simulink model "proj_lqr"  (R2021a)
settings: Solver=VariableStepAuto  StartTime=0.0  StopTime=400  RelTol=1e-3
values from neighbouring files (symbols this model uses):
  A = [0 0 1 0 ... (first row only)    [proj_LQRcode.m]    (also in proj_PIDcode.m)
  B = [0 0 ... (first row only)    [proj_LQRcode.m]    (also in proj_PIDcode.m)
  C = [1 0 0 0 ... (first row only)    [proj_LQRcode.m]    (also in proj_PIDcode.m)
  K = lqr(A,B,Q,R)    [proj_LQRcode.m]
  L = lqr(A',C',QB,RB)'    [proj_LQRcode.m]
  x0 = [-3.1;-39.16;0.00002;0.0041]    [proj_LQRcode.m]
settings Model: Creator=huangzijing  LastModifiedBy=huangzijing

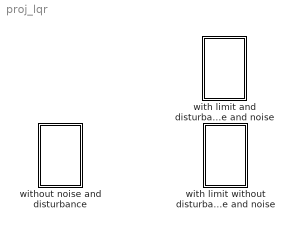
== system proj_lqr ==
  with limit and disturbance and noise : Subsystem
  "with limit without disturbance and noise " : Subsystem
  without noise and disturbance : Subsystem

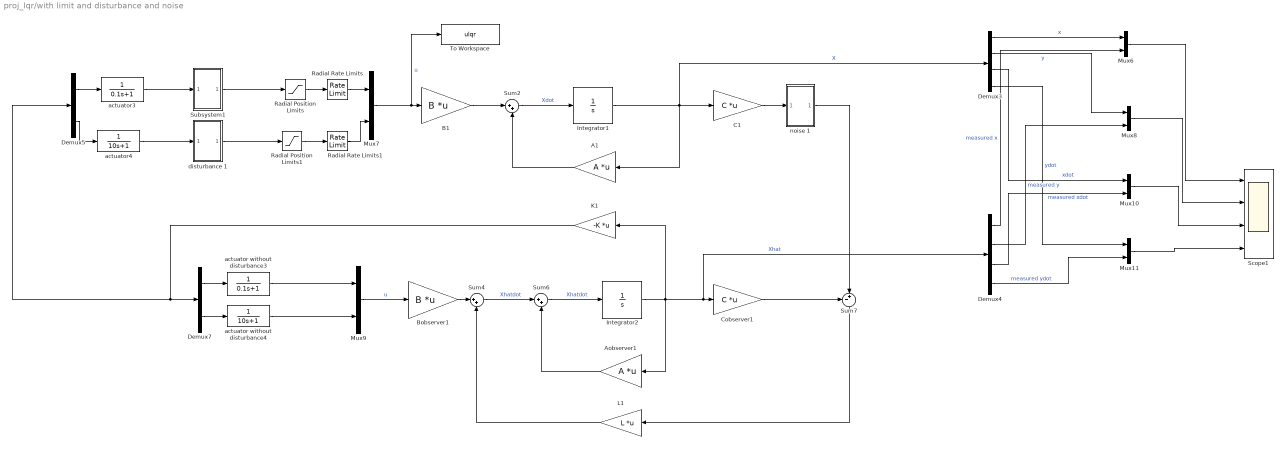
== system proj_lqr/with limit and disturbance and noise ==
  A1 : Gain  Gain=A  Multiplication=Matrix(K*u)
  Aobserver1 : Gain  Gain=A  Multiplication=Matrix(K*u)
  B1 : Gain  Gain=B  Multiplication=Matrix(K*u)
  Bobserver1 : Gain  Gain=B  Multiplication=Matrix(K*u)
  C1 : Gain  Gain=C  Multiplication=Matrix(K*u)
  Cobserver1 : Gain  Gain=C  Multiplication=Matrix(K*u)
  Demux3 : Demux
  Demux4 : Demux
  Demux5 : Demux  Outputs=2
  Demux7 : Demux  Outputs=2
  Integrator1 : Integrator  InitialCondition=x0
  Integrator2 : Integrator  InitialCondition=x0
  K1 : Gain  Gain=-K  Multiplication=Matrix(K*u)
  L1 : Gain  Gain=L  Multiplication=Matrix(K*u)
  Mux{6..11} (6 alike) : Mux  Inputs=2
  Radial Position Limits : Saturate  UpperLimit=5880  LowerLimit=-5880
  Radial Position Limits1 : Saturate  UpperLimit=5880  LowerLimit=-5880
  Radial Rate Limits : RateLimiter  RisingSlewLimit=30  FallingSlewLimit=-30  SampleTimeMode=inherited
  Radial Rate Limits1 : RateLimiter  RisingSlewLimit=30  FallingSlewLimit=-30  SampleTimeMode=inherited
  Scope1 : Scope  NumInputPorts=4
  Subsystem1 : Subsystem
  Sum2 : Sum  Inputs=|++
  Sum4 : Sum  Inputs=|++
  Sum6 : Sum  Inputs=|++
  Sum7 : Sum  Inputs=-+|
  To Workspace : ToWorkspace  VariableName=ulqr  SampleTime=-1
      settings: Save2DSignal=2-D array (concatenate along first dimension)
  actuator without disturbance3 : TransferFcn  Denominator=[0.1 1]
  actuator without disturbance4 : TransferFcn  Denominator=[10 1]
  actuator3 : TransferFcn  Denominator=[0.1 1]
  actuator4 : TransferFcn  Denominator=[10 1]
  disturbance 1 : Subsystem
  noise 1 : Subsystem
  wires:
  actuator without disturbance4/1 -> Mux9/2
  Demux7/2 -> actuator without disturbance4/1
  Demux4/4 -> Mux11/2  "measured ydot"
  Radial Rate Limits1/1 -> Mux7/2
  A1/1 -> Sum2/2
  Aobserver1/1 -> Sum6/2
  Demux4/2 -> Mux8/2  "measured y"
  Demux4/3 -> Mux10/2  "measured xdot"
  Cobserver1/1 -> Sum7/1
  Mux9/1 -> Bobserver1/1  "u"
  Integrator1/1 -> A1/1, C1/1, Demux3/1  "X"
  Demux3/1 -> Mux6/1  "x"
  Bobserver1/1 -> Sum4/1
  Mux6/1 -> Scope1/1
  Demux3/3 -> Mux10/1  "xdot"
  Demux4/1 -> Mux6/2  "measured x"
  Demux7/1 -> actuator without disturbance3/1
  K1/1 -> Demux5/1, Demux7/1
  Demux5/1 -> actuator3/1
  Integrator2/1 -> Demux4/1, Cobserver1/1, K1/1, Aobserver1/1  "Xhat"
  Radial Position Limits1/1 -> Radial Rate Limits1/1
  Demux3/4 -> Mux11/1  "ydot"
  Mux8/1 -> Scope1/2
  Demux3/2 -> Mux8/1  "y"
  L1/1 -> Sum4/2
  Mux7/1 -> To Workspace/1, B1/1  "u"
  Sum2/1 -> Integrator1/1  "Xdot"
  Radial Position Limits/1 -> Radial Rate Limits/1
  Demux5/2 -> actuator4/1
  Mux11/1 -> Scope1/4
  Sum6/1 -> Integrator2/1  "Xhatdot"
  Mux10/1 -> Scope1/3
  Sum7/1 -> L1/1
  B1/1 -> Sum2/1
  Sum4/1 -> Sum6/1  "Xhatdot"
  Radial Rate Limits/1 -> Mux7/1
  actuator without disturbance3/1 -> Mux9/1
  actuator3/1 -> Subsystem1/1(In1)
  Subsystem1/1(Out1) -> Radial Position Limits/1
  disturbance 1/1(Out1) -> Radial Position Limits1/1
  actuator4/1 -> disturbance 1/1(In1)
  C1/1 -> noise 1/1(In1)
  noise 1/1(Out1) -> Sum7/2

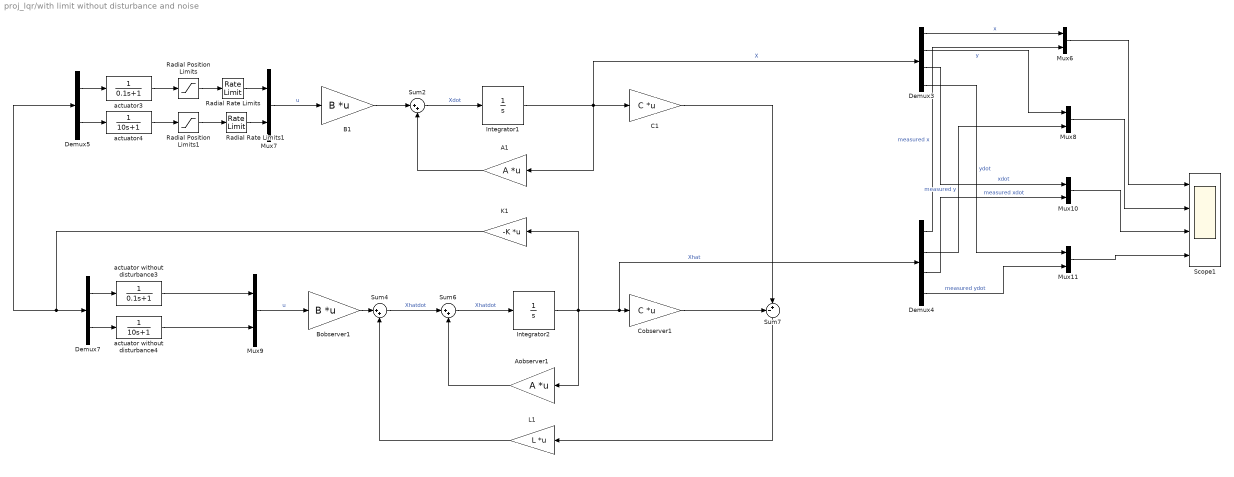
== system proj_lqr/with limit without disturbance and noise  ==
  A1 : Gain  Gain=A  Multiplication=Matrix(K*u)
  Aobserver1 : Gain  Gain=A  Multiplication=Matrix(K*u)
  B1 : Gain  Gain=B  Multiplication=Matrix(K*u)
  Bobserver1 : Gain  Gain=B  Multiplication=Matrix(K*u)
  C1 : Gain  Gain=C  Multiplication=Matrix(K*u)
  Cobserver1 : Gain  Gain=C  Multiplication=Matrix(K*u)
  Demux3 : Demux
  Demux4 : Demux
  Demux5 : Demux  Outputs=2
  Demux7 : Demux  Outputs=2
  Integrator1 : Integrator  InitialCondition=x0
  Integrator2 : Integrator  InitialCondition=x0
  K1 : Gain  Gain=-K  Multiplication=Matrix(K*u)
  L1 : Gain  Gain=L  Multiplication=Matrix(K*u)
  Mux{6..11} (6 alike) : Mux  Inputs=2
  Radial Position Limits : Saturate  UpperLimit=5880  LowerLimit=-5880
  Radial Position Limits1 : Saturate  UpperLimit=5880  LowerLimit=-5880
  Radial Rate Limits : RateLimiter  RisingSlewLimit=30  FallingSlewLimit=-30  SampleTimeMode=inherited
  Radial Rate Limits1 : RateLimiter  RisingSlewLimit=30  FallingSlewLimit=-30  SampleTimeMode=inherited
  Scope1 : Scope  NumInputPorts=4
  Sum2 : Sum  Inputs=|++
  Sum4 : Sum  Inputs=|++
  Sum6 : Sum  Inputs=|++
  Sum7 : Sum  Inputs=-+|
  actuator without disturbance3 : TransferFcn  Denominator=[0.1 1]
  actuator without disturbance4 : TransferFcn  Denominator=[10 1]
  actuator3 : TransferFcn  Denominator=[0.1 1]
  actuator4 : TransferFcn  Denominator=[10 1]
  wires:
  C1/1 -> Sum7/2
  Demux3/1 -> Mux6/1  "x"
  Bobserver1/1 -> Sum4/1
  Demux4/1 -> Mux6/2  "measured x"
  Sum2/1 -> Integrator1/1  "Xdot"
  Mux9/1 -> Bobserver1/1  "u"
  A1/1 -> Sum2/2
  K1/1 -> Demux5/1, Demux7/1
  Demux4/3 -> Mux10/2  "measured xdot"
  Mux8/1 -> Scope1/2
  Demux5/2 -> actuator4/1
  Mux11/1 -> Scope1/4
  Integrator1/1 -> A1/1, C1/1, Demux3/1  "X"
  Demux4/4 -> Mux11/2  "measured ydot"
  Demux3/4 -> Mux11/1  "ydot"
  Demux3/2 -> Mux8/1  "y"
  Demux5/1 -> actuator3/1
  Demux7/1 -> actuator without disturbance3/1
  L1/1 -> Sum4/2
  Mux10/1 -> Scope1/3
  Sum4/1 -> Sum6/1  "Xhatdot"
  Cobserver1/1 -> Sum7/1
  Sum7/1 -> L1/1
  B1/1 -> Sum2/1
  Sum6/1 -> Integrator2/1  "Xhatdot"
  Demux4/2 -> Mux8/2  "measured y"
  Mux6/1 -> Scope1/1
  Demux7/2 -> actuator without disturbance4/1
  Integrator2/1 -> Demux4/1, Cobserver1/1, K1/1, Aobserver1/1  "Xhat"
  Aobserver1/1 -> Sum6/2
  Demux3/3 -> Mux10/1  "xdot"
  Mux7/1 -> B1/1  "u"
  actuator3/1 -> Radial Position Limits/1
  Radial Position Limits/1 -> Radial Rate Limits/1
  Radial Rate Limits/1 -> Mux7/1
  actuator4/1 -> Radial Position Limits1/1
  Radial Position Limits1/1 -> Radial Rate Limits1/1
  Radial Rate Limits1/1 -> Mux7/2
  actuator without disturbance3/1 -> Mux9/1
  actuator without disturbance4/1 -> Mux9/2

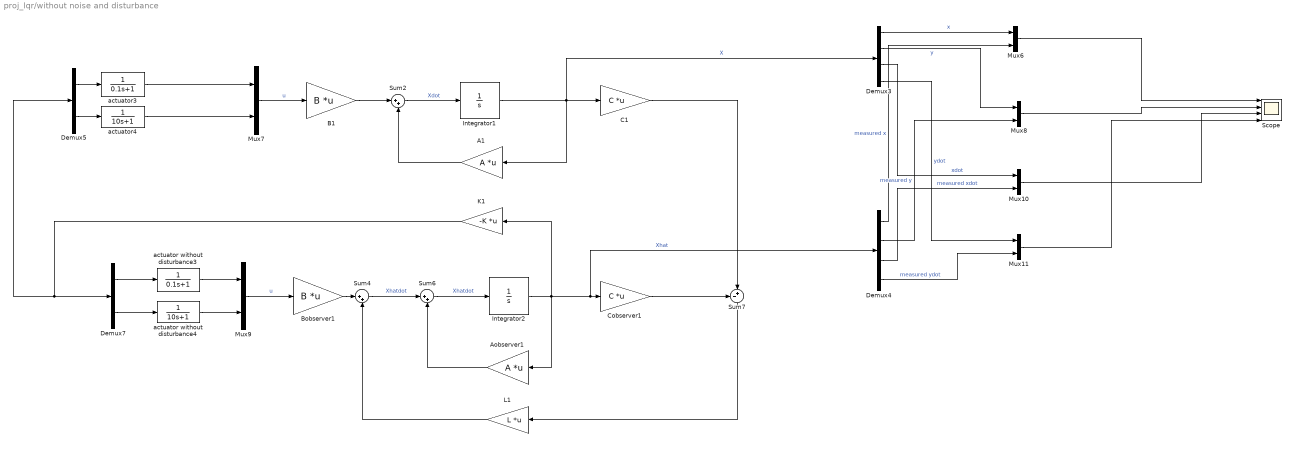
== system proj_lqr/without noise and disturbance ==
  A1 : Gain  Gain=A  Multiplication=Matrix(K*u)
  Aobserver1 : Gain  Gain=A  Multiplication=Matrix(K*u)
  B1 : Gain  Gain=B  Multiplication=Matrix(K*u)
  Bobserver1 : Gain  Gain=B  Multiplication=Matrix(K*u)
  C1 : Gain  Gain=C  Multiplication=Matrix(K*u)
  Cobserver1 : Gain  Gain=C  Multiplication=Matrix(K*u)
  Demux3 : Demux
  Demux4 : Demux
  Demux5 : Demux  Outputs=2
  Demux7 : Demux  Outputs=2
  Integrator1 : Integrator  InitialCondition=x0
  Integrator2 : Integrator  InitialCondition=x0
  K1 : Gain  Gain=-K  Multiplication=Matrix(K*u)
  L1 : Gain  Gain=L  Multiplication=Matrix(K*u)
  Mux{6..11} (6 alike) : Mux  Inputs=2
  Scope : Scope  NumInputPorts=4
  Sum2 : Sum  Inputs=|++
  Sum4 : Sum  Inputs=|++
  Sum6 : Sum  Inputs=|++
  Sum7 : Sum  Inputs=-+|
  actuator without disturbance3 : TransferFcn  Denominator=[0.1 1]
  actuator without disturbance4 : TransferFcn  Denominator=[10 1]
  actuator3 : TransferFcn  Denominator=[0.1 1]
  actuator4 : TransferFcn  Denominator=[10 1]
  wires:
  C1/1 -> Sum7/2
  Demux3/1 -> Mux6/1  "x"
  Bobserver1/1 -> Sum4/1
  Demux4/1 -> Mux6/2  "measured x"
  Sum2/1 -> Integrator1/1  "Xdot"
  Mux9/1 -> Bobserver1/1  "u"
  A1/1 -> Sum2/2
  K1/1 -> Demux5/1, Demux7/1
  Demux4/3 -> Mux10/2  "measured xdot"
  Demux5/2 -> actuator4/1
  Integrator1/1 -> A1/1, C1/1, Demux3/1  "X"
  Demux4/4 -> Mux11/2  "measured ydot"
  Demux3/4 -> Mux11/1  "ydot"
  Demux3/2 -> Mux8/1  "y"
  Demux5/1 -> actuator3/1
  Demux7/1 -> actuator without disturbance3/1
  actuator without disturbance4/1 -> Mux9/2
  L1/1 -> Sum4/2
  actuator3/1 -> Mux7/1
  Mux10/1 -> Scope/3
  Sum4/1 -> Sum6/1  "Xhatdot"
  Cobserver1/1 -> Sum7/1
  Sum7/1 -> L1/1
  B1/1 -> Sum2/1
  Sum6/1 -> Integrator2/1  "Xhatdot"
  Demux4/2 -> Mux8/2  "measured y"
  Mux6/1 -> Scope/1
  Demux7/2 -> actuator without disturbance4/1
  actuator4/1 -> Mux7/2
  Integrator2/1 -> Demux4/1, Cobserver1/1, K1/1, Aobserver1/1  "Xhat"
  Aobserver1/1 -> Sum6/2
  Demux3/3 -> Mux10/1  "xdot"
  Mux7/1 -> B1/1  "u"
  actuator without disturbance3/1 -> Mux9/1
  Mux8/1 -> Scope/2
  Mux11/1 -> Scope/4

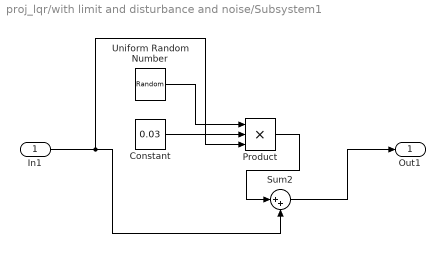
== system proj_lqr/with limit and disturbance and noise/Subsystem1 ==
  In1 : Inport
  Constant : Constant  Value=0.03
  Product : Product  Inputs=3
  Sum2 : Sum  Inputs=|++
  Uniform Random Number : UniformRandomNumber  SampleTime=0.1
  Out1 : Outport
  wires:
  Sum2/1 -> Out1/1
  Constant/1 -> Product/2
  Uniform Random Number/1 -> Product/1
  In1/1 -> Sum2/2, Product/3
  Product/1 -> Sum2/1

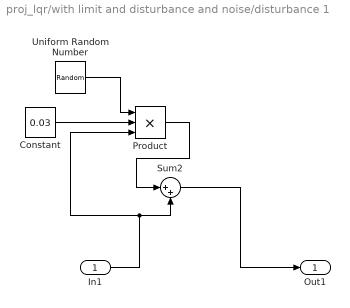
== system proj_lqr/with limit and disturbance and noise/disturbance 1 ==
  In1 : Inport
  Constant : Constant  Value=0.03
  Product : Product  Inputs=3
  Sum2 : Sum  Inputs=|++
  Uniform Random Number : UniformRandomNumber  SampleTime=0.1
  Out1 : Outport
  wires:
  Constant/1 -> Product/2
  Uniform Random Number/1 -> Product/1
  Sum2/1 -> Out1/1
  In1/1 -> Sum2/2, Product/3
  Product/1 -> Sum2/1

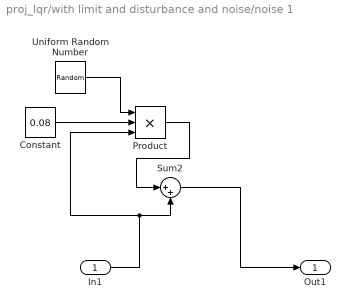
== system proj_lqr/with limit and disturbance and noise/noise 1 ==
  In1 : Inport
  Constant : Constant  Value=0.08
  Product : Product  Inputs=3
  Sum2 : Sum  Inputs=|++
  Uniform Random Number : UniformRandomNumber  SampleTime=0.1
  Out1 : Outport
  wires:
  Constant/1 -> Product/2
  Uniform Random Number/1 -> Product/1
  Sum2/1 -> Out1/1
  In1/1 -> Sum2/2, Product/3
  Product/1 -> Sum2/1
